simulink model "GeneralQuadrotorKinetics"  (R2022b)
settings: Solver=ode4  StartTime=0.0  StopTime=10.0  FixedStep=0.001  RelTol=1e-3
libraries: matrix_library x1
settings Model: Creator=Baoyi Cui  LastModifiedBy=Baoyi Cui

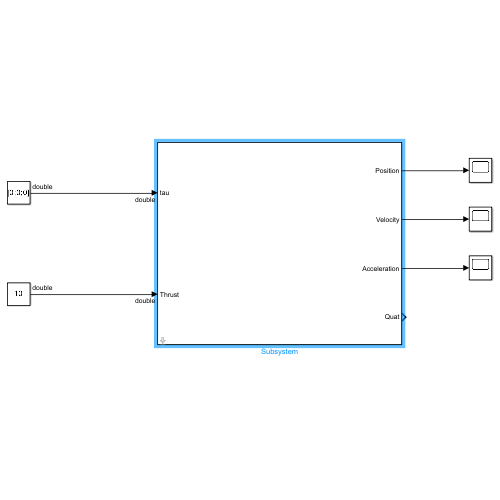
[thumbnail: Simulink's stored preview of the top-level diagram]
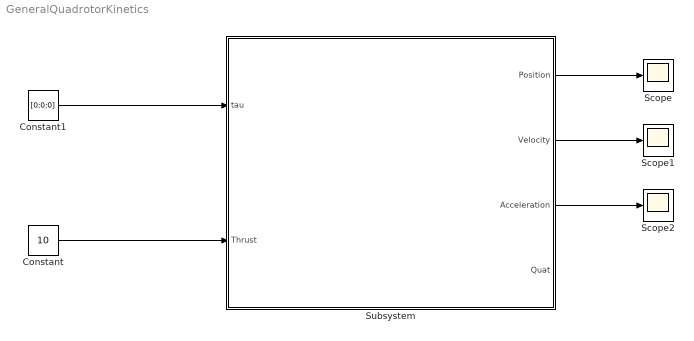
== system GeneralQuadrotorKinetics ==
  Constant : Constant  Value=10
  Constant1 : Constant  Value=[0;0;0]
  Scope : Scope
  Scope1 : Scope
  Scope2 : Scope
  Subsystem : Subsystem  mask{m=1, Ixx=0.006721, Iyy=0.008041, Izz=0.014279, g=9.8, rotorDragCoeff=diag([0, 0, 0]), kh=0, InitialPosition=[0; 0; 0], InitialVelocity=[0;0;0], InitialAttitude=[1,0,0,0], IntialAngularVelocity=[0; 0; 0]}
      mask prompts: m "无人机质量(kg)"; Ixx "x轴转动惯量(kg*m^2)"; Iyy "y轴转动惯量(kg*m^2)"; Izz "z轴转动惯量(kg*m^2)"; g "重力加速度(m/s^2)"; rotorDragCoeff "rotor-drag系数"; kh "水平阻力系数"; InitialPosition "初始位置(m)"; InitialVelocity "初始速度(m/s)"; InitialAttitude "初始姿态(qw, qx, qy, qz)"; IntialAngularVelocity "初始角速度"
      mask DialogControl ParameterGroupVar Prompt: 参数
  wires:
  Constant/1 -> Subsystem/2(Thrust)
  Constant1/1 -> Subsystem/1(tau)
  Subsystem/1(Position) -> Scope/1
  Subsystem/2(Velocity) -> Scope1/1
  Subsystem/3(Acceleration) -> Scope2/1

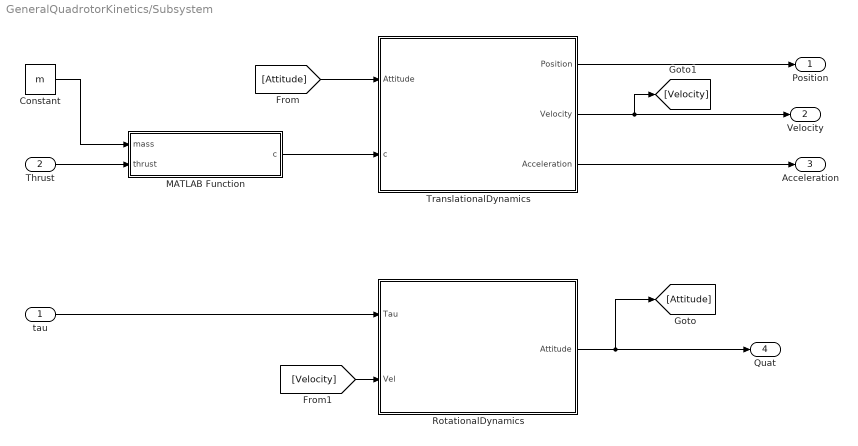
== system GeneralQuadrotorKinetics/Subsystem ==
  tau : Inport
  Thrust : Inport  Port=2
  Constant : Constant  Value=m
  MATLAB Function : MATLAB Function  TreatAsAtomicUnit=on
  RotationalDynamics : Subsystem
  TranslationalDynamics : Subsystem
  Position : Outport
  Velocity : Outport  Port=2
  Acceleration : Outport  Port=3
  Quat : Outport  Port=4
  wires:
  Thrust/1 -> MATLAB Function/2(thrust)
  MATLAB Function/1(c) -> TranslationalDynamics/2(c)
  RotationalDynamics/1(Attitude) -> Quat/1, [Attitude]
  [Attitude] -> TranslationalDynamics/1(Attitude)
  TranslationalDynamics/1(Position) -> Position/1
  TranslationalDynamics/2(Velocity) -> Velocity/1, [Velocity]
  TranslationalDynamics/3(Acceleration) -> Acceleration/1
  [Velocity] -> RotationalDynamics/2(Vel)
  tau/1 -> RotationalDynamics/1(Tau)
  Constant/1 -> MATLAB Function/1(mass)

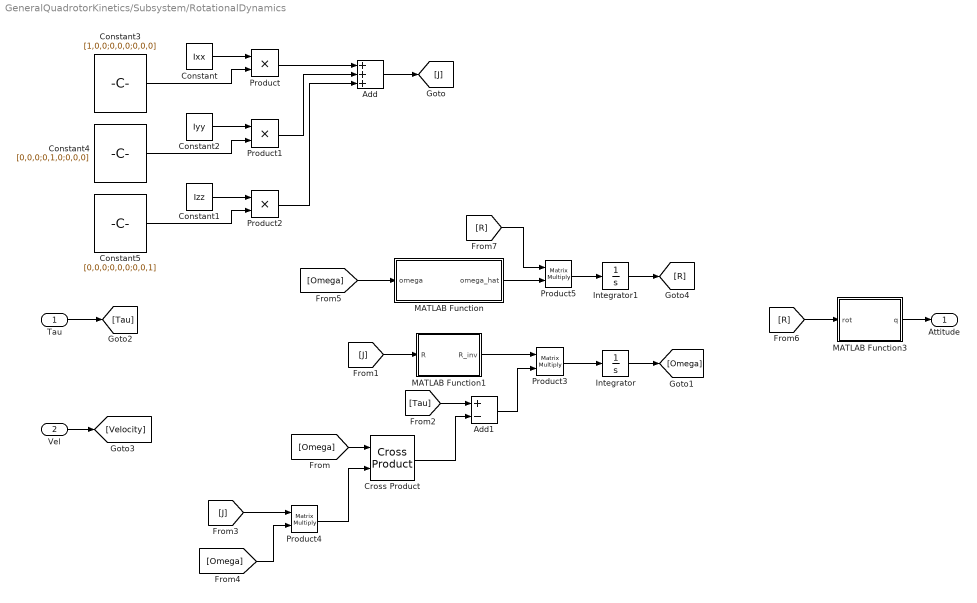
== system GeneralQuadrotorKinetics/Subsystem/RotationalDynamics ==
  Tau : Inport
  Vel : Inport  Port=2
  Add : Sum  Inputs=+++
  Add1 : Sum  Inputs=+-
  Constant : Constant  Value=Ixx
  Constant1 : Constant  Value=Izz
  Constant2 : Constant  Value=Iyy
  Constant3 : Constant  Value=[1,0,0;0,0,0;0,0,0]
  Constant4 : Constant  Value=[0,0,0;0,1,0;0,0,0]
  Constant5 : Constant  Value=[0,0,0;0,0,0;0,0,1]
  Cross Product : matrix_library/Cross Product
  Integrator : Integrator  InitialCondition=[0;0;0]
  Integrator1 : Integrator
  MATLAB Function : MATLAB Function  TreatAsAtomicUnit=on
  MATLAB Function1 : MATLAB Function  TreatAsAtomicUnit=on
  MATLAB Function3 : MATLAB Function  TreatAsAtomicUnit=on
  Product : Product
  Product1 : Product
  Product2 : Product
  Product3 : Product  Multiplication=Matrix(*)
  Product4 : Product  Multiplication=Matrix(*)
  Product5 : Product  Multiplication=Matrix(*)
  Attitude : Outport
  wires:
  Constant/1 -> Product/1
  Constant2/1 -> Product1/1
  Constant1/1 -> Product2/1
  Constant3/1 -> Product/2
  Constant4/1 -> Product1/2
  Constant5/1 -> Product2/2
  Product/1 -> Add/1
  Product1/1 -> Add/2
  Product2/1 -> Add/3
  Add/1 -> [J]
  [J] -> MATLAB Function1/1(R)
  MATLAB Function1/1(R_inv) -> Product3/1
  Tau/1 -> [Tau]
  Vel/1 -> [Velocity]
  [Tau] -> Add1/1
  [Omega] -> Cross Product/1
  [J] -> Product4/1
  [Omega] -> Product4/2
  Product4/1 -> Cross Product/2
  Cross Product/1 -> Add1/2
  Add1/1 -> Product3/2
  Product3/1 -> Integrator/1
  Integrator/1 -> [Omega]
  [Omega] -> MATLAB Function/1(omega)
  MATLAB Function/1(omega_hat) -> Product5/2
  Product5/1 -> Integrator1/1
  Integrator1/1 -> [R]
  [R] -> MATLAB Function3/1(rot)
  MATLAB Function3/1(q) -> Attitude/1
  [R] -> Product5/1

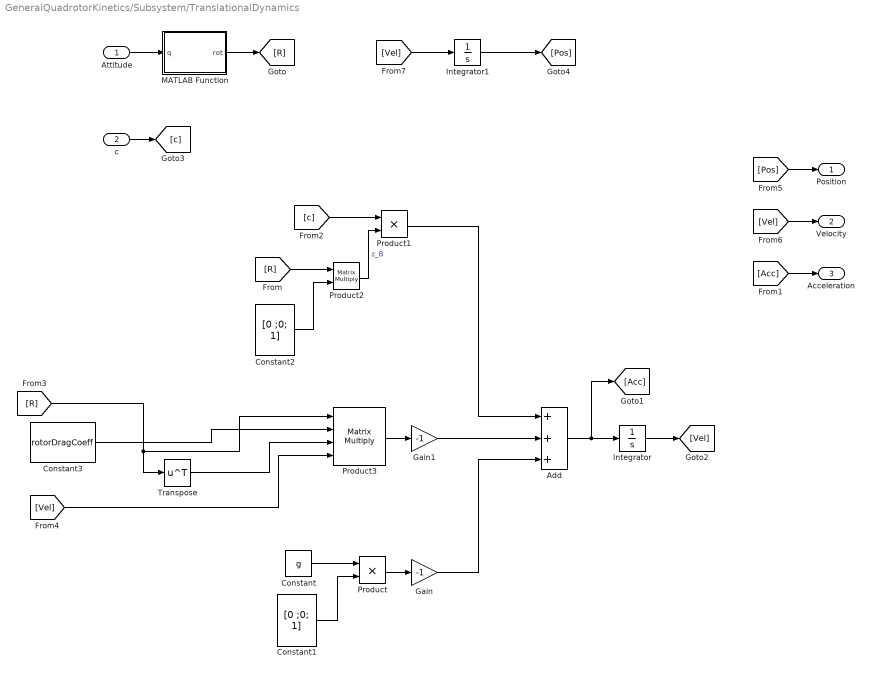
== system GeneralQuadrotorKinetics/Subsystem/TranslationalDynamics ==
  Attitude : Inport
  c : Inport  Port=2
  Add : Sum  Inputs=+++
  Constant : Constant  Value=g
  Constant1 : Constant  Value=[0 ;0; 1]  VectorParams1D=off
  Constant2 : Constant  Value=[0 ;0; 1]  VectorParams1D=off
  Constant3 : Constant  Value=rotorDragCoeff
  Gain : Gain  Gain=-1
  Gain1 : Gain  Gain=-1
  Integrator : Integrator  InitialCondition=InitialVelocity
  Integrator1 : Integrator  InitialCondition=InitialPosition
  MATLAB Function : MATLAB Function  TreatAsAtomicUnit=on
  Product : Product
  Product1 : Product
  Product2 : Product  Multiplication=Matrix(*)
  Product3 : Product  Inputs=4  Multiplication=Matrix(*)
  Transpose : Math  Operator=transpose
  Position : Outport
  Velocity : Outport  Port=2
  Acceleration : Outport  Port=3
  wires:
  Attitude/1 -> MATLAB Function/1(q)
  MATLAB Function/1(rot) -> [R]
  Constant/1 -> Product/1
  Constant1/1 -> Product/2
  Product/1 -> Gain/1
  [Acc] -> Acceleration/1
  Add/1 -> [Acc], Integrator/1
  Integrator/1 -> [Vel]
  Gain/1 -> Add/3
  c/1 -> [c]
  [c] -> Product1/1
  [R] -> Product2/1
  Constant2/1 -> Product2/2
  Product2/1 -> Product1/2  "z_B"
  Product1/1 -> Add/1
  [R] -> Product3/1, Transpose/1
  Product3/1 -> Gain1/1
  Gain1/1 -> Add/2
  Constant3/1 -> Product3/2
  Transpose/1 -> Product3/3
  [Vel] -> Product3/4
  [Vel] -> Integrator1/1
  [Vel] -> Velocity/1
  [Pos] -> Position/1
  Integrator1/1 -> [Pos]

== matlab function GeneralQuadrotorKinetics/Subsystem/TranslationalDynamics/MATLAB Function ==
  data: q input; rot output
function rot = quat2rotMat(q)
    rot = quat2dcm(quatnormalize(q));

== matlab function GeneralQuadrotorKinetics/Subsystem/RotationalDynamics/MATLAB Function ==
  data: omega input; omega_hat output
function omega_hat = getSkewSymmetricMat(omega)
    omega_hat = zeros(3,3);
    omega_x = omega(1);
    omega_y = omega(2);
    omega_z = omega(3);
    omega_hat(1,2) = -omega_z;
    omega_hat(1,3) = omega_y;
    omega_hat(2,1) = omega_z;
    omega_hat(2,3) = -omega_x;
    omega_hat(3,1) = -omega_y;
    omega_hat(3,2) = omega_x;

== matlab function GeneralQuadrotorKinetics/Subsystem/RotationalDynamics/MATLAB Function1 ==
  data: R input; R_inv output
function R_inv = getInvMat(R)
    R_inv = inv(R);

== matlab function GeneralQuadrotorKinetics/Subsystem/RotationalDynamics/MATLAB Function3 ==
  data: rot input; q output
function q = quat2rotMat(rot)
    q = [1;0;0;0];
    q = dcm2quat(rot);

== matlab function GeneralQuadrotorKinetics/Subsystem/MATLAB Function ==
  data: mass input; thrust input; c output
function c = thrustNomalization(mass, thrust)
    c = thrust / mass;
